simulink model "Comparingstatespaceandtransferfunction2"  (R2019b)
settings: Solver=VariableStepAuto  StartTime=0.0  StopTime=10.0  RelTol=1e-3
undefined symbols (not defined in the file or in its folder): b, k
settings Model: Creator=marslab  LastModifiedBy=marslab

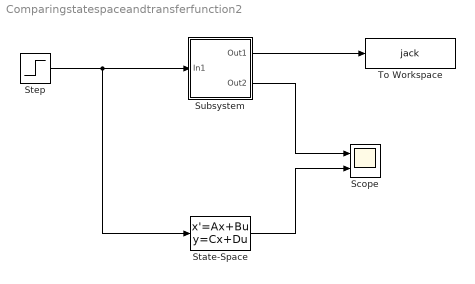
== system Comparingstatespaceandtransferfunction2 ==
  Scope : Scope  NumInputPorts=2
  State-Space : StateSpace  A=[0 1;-k -b]  B=[0 ;1]  C=[1 0]  D=0  InitialCondition=0
  Step : Step  SampleTime=0.1
  Subsystem : Subsystem
  To Workspace : ToWorkspace  VariableName=jack  SaveFormat=Timeseries  SampleTime=-1
  wires:
  Subsystem/1(Out1) -> To Workspace/1
  Subsystem/2(Out2) -> Scope/1
  Step/1 -> State-Space/1, Subsystem/1(In1)
  State-Space/1 -> Scope/2

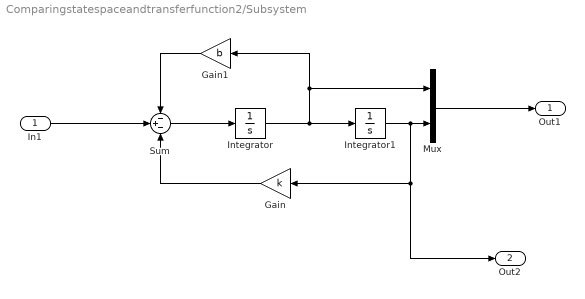
== system Comparingstatespaceandtransferfunction2/Subsystem ==
  In1 : Inport
  Gain : Gain  Gain=k
  Gain1 : Gain  Gain=b
  Integrator : Integrator
  Integrator1 : Integrator
  Mux : Mux  Inputs=2
  Sum : Sum  Inputs=-+-
  Out1 : Outport
  Out2 : Outport  Port=2
  wires:
  Integrator/1 -> Gain1/1, Mux/1, Integrator1/1
  Gain/1 -> Sum/3
  In1/1 -> Sum/2
  Gain1/1 -> Sum/1
  Integrator1/1 -> Mux/2, Out2/1, Gain/1
  Sum/1 -> Integrator/1
  Mux/1 -> Out1/1
